simulink model "signal_bruite"  (R2019b)
settings: Solver=FixedStepAuto  StartTime=0.0  StopTime=25  FixedStep=0.001  RelTol=1e-3
undefined symbols (not defined in the file): sigbuilder_block
settings Model: Creator=Ivan  LastModifiedBy=ivanl
settings SFSimCC: CustomCodeUndefinedFunction=UseInterfaceOnly

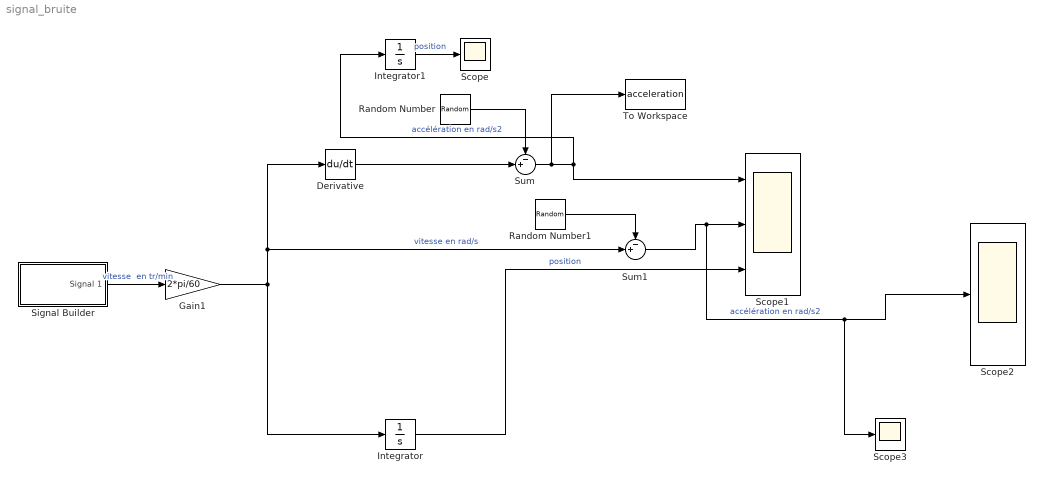
== system signal_bruite ==
  Derivative : Derivative  CoefficientInTFapproximation=0.01
  Gain1 : Gain  Gain=2*pi/60
  Integrator : Integrator
  Integrator1 : Integrator
  Random Number : RandomNumber  Variance=0.8  Seed=10  SampleTime=0.01
  Random Number1 : RandomNumber  Variance=0.8  SampleTime=0.01
  Scope : Scope
  Scope1 : Scope  NumInputPorts=3
  Scope2 : Scope
  Scope3 : Scope
  Signal Builder : Subsystem  Tag=STV Subsys  LoadFcn=sigbuilder_block('load');  StartFcn=sigbuilder_block('start');  StopFcn=sigbuilder_block('stop');  ClipboardFcn=sigbuilder_block('clipboard');  mask(Sigbuilder block){tuvar=[0:10]}
      mask help: Simulink:masks:SigbuilderBlock_MD
      mask init:
      | if ~strcmp(get_param(bdroot(gcbh),'SimulationStatus'),'stopped') tuvar = sigbuilder_block('maskInit'); end
      settings: CopyFcn=sigbuilder_block('copy');  DeleteFcn=sigbuilder_block('delete');  ModelCloseFcn=sigbuilder_block('modelClose');  PreSaveFcn=sigbuilder_block('preSave');  PauseFcn=sigbuilder_block('pause');  ContinueFcn=sigbuilder_block('continue');  NameChangeFcn=sigbuilder_block('namechange');  OpenFcn=sigbuilder_block('open',[536.25 206.25 550.5 399.75 ]);  CloseFcn=sigbuilder_block('close');
      mask Display: plot(0, 0, 100, 100,[2, 2, 32, 32, 2], [68, 8, 8, 68, 68],[32, 2], [38, 38], [32, 19, 2],[53, 60, 44], [32, 17, 17, 2],[16, 16, 31, 31]);txt = getActiveGroup(gcbh);text(2, 100, txt,'verticalAlignment', 'top');
  Sum : Sum  Inputs=-+|
  Sum1 : Sum  Inputs=-+|
  To Workspace : ToWorkspace  VariableName=acceleration  SampleTime=-1
  wires:
  Signal Builder/1(Signal 1) -> Gain1/1  "vitesse  en tr/min"
  Integrator/1 -> Scope1/3  "position"
  Random Number/1 -> Sum/1
  Sum/1 -> To Workspace/1, Integrator1/1, Scope1/1  "accélération en rad/s2"
  Gain1/1 -> Derivative/1, Sum1/2, Integrator/1  "vitesse en rad/s"
  Derivative/1 -> Sum/2
  Integrator1/1 -> Scope/1  "position"
  Sum1/1 -> Scope3/1, Scope2/1, Scope1/2  "accélération en rad/s2"
  Random Number1/1 -> Sum1/1

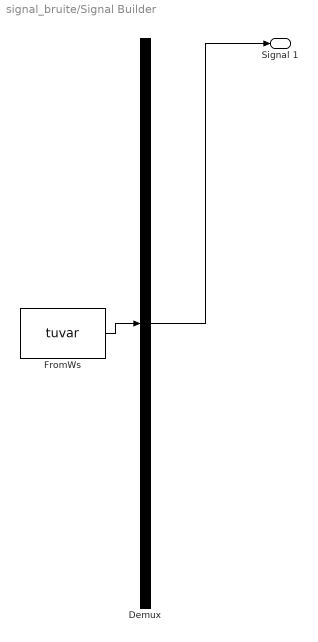
== system signal_bruite/Signal Builder ==
  Demux : Demux  Tag=STV Demux  Outputs=1
  FromWs : FromWorkspace  Tag=STV FromWs  VariableName=tuvar  SampleTime=0
      SigBuilderData=|
      | common.afterFinalStr = 'Extrapolate'
      | common.sampleTime = 0
      | dataSet.timeRange = [0 25]
      | dataSet.name = 'Group 1'
      | sbobj.Groups.Name = 'Group 1'
      | sbobj.Groups.Signals.Name = 'Signal 1'
      | sbobj.Groups.Signals.XData = [0 1 3 15 20 25]
      | sbobj.Groups.Signals.YData = [0 0 250 250 0 0]
      | sbobj.Groups.TimeRange = [0 25]
  Signal 1 : Outport  Tag=STV Outport  VectorParamsAs1DForOutWhenUnconnected=off
  wires:
  Demux/1 -> Signal 1/1
  FromWs/1 -> Demux/1
